simulink model "sim_tire_model"  (R2014b)
settings: Solver=ode45  StartTime=0.0  StopTime=10.0  RelTol=1e-3
settings Model: Creator=Kevin  LastModifiedBy=Kevin

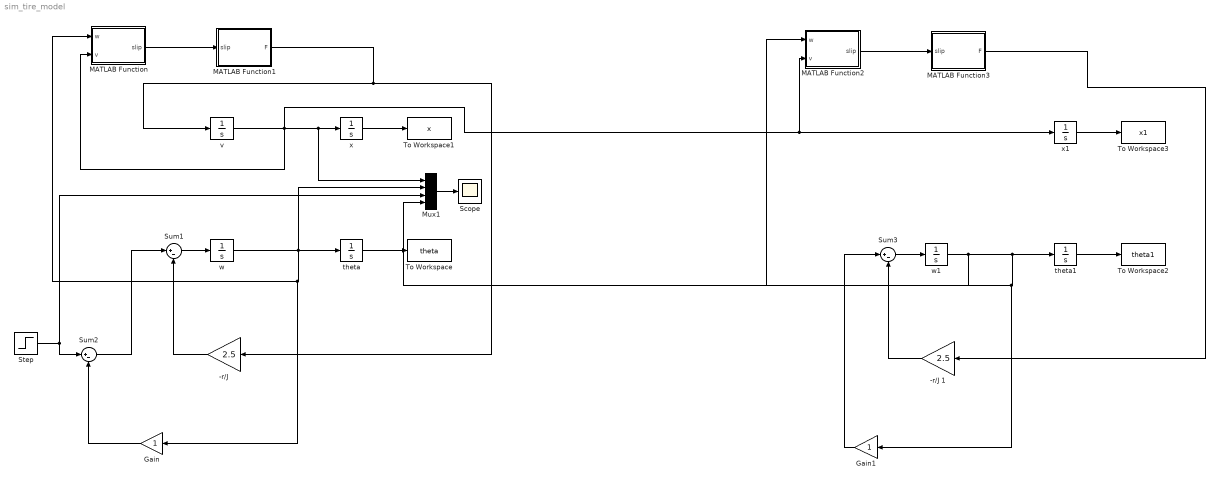
== system sim_tire_model ==
  "-r/J " : Gain  Gain=2.5
  -r/J 1 : Gain  Gain=2.5
  Gain : Gain
  Gain1 : Gain
  MATLAB Function : MATLAB Function  TreatAsAtomicUnit=on
  MATLAB Function1 : MATLAB Function  TreatAsAtomicUnit=on
  MATLAB Function2 : MATLAB Function  TreatAsAtomicUnit=on
  MATLAB Function3 : MATLAB Function  TreatAsAtomicUnit=on
  Mux1 : Mux
  Scope : Scope
      settings: ShowLegends=on
  Step : Step  Before=5  After=0  SampleTime=0
  Sum1 : Sum  Inputs=|+-
  Sum2 : Sum  Inputs=|+-
  Sum3 : Sum  Inputs=|+-
  To Workspace : ToWorkspace  VariableName=theta  SampleTime=-1
      settings: Decimation=2  Save2DSignal=2-D array (concatenate along first dimension)
  To Workspace1 : ToWorkspace  VariableName=x  SampleTime=-1
      settings: Decimation=2  Save2DSignal=2-D array (concatenate along first dimension)
  To Workspace2 : ToWorkspace  VariableName=theta1  SampleTime=-1
      settings: Decimation=2  Save2DSignal=2-D array (concatenate along first dimension)
  To Workspace3 : ToWorkspace  VariableName=x1  SampleTime=-1
      settings: Decimation=2  Save2DSignal=2-D array (concatenate along first dimension)
  theta : Integrator
  theta1 : Integrator
  "v " : Integrator
  w : Integrator
  w1 : Integrator
  x : Integrator
  x1 : Integrator
  wires:
  w/1 -> Mux1/2, Gain/1, MATLAB Function/1(w), theta/1
  "v "/1 -> MATLAB Function2/2(v), x1/1, MATLAB Function/2(v), Mux1/1, x/1
  MATLAB Function1/1(F) -> "-r/J "/1, "v "/1
  Sum1/1 -> w/1
  "-r/J "/1 -> Sum1/2
  MATLAB Function/1(slip) -> MATLAB Function1/1(slip)
  Step/1 -> Mux1/3, Sum2/1
  Sum2/1 -> Sum1/1
  Gain/1 -> Sum2/2
  theta/1 -> To Workspace/1
  x/1 -> To Workspace1/1
  MATLAB Function3/1(F) -> -r/J 1/1
  Sum3/1 -> w1/1
  -r/J 1/1 -> Sum3/2
  MATLAB Function2/1(slip) -> MATLAB Function3/1(slip)
  Gain1/1 -> Sum3/1
  theta1/1 -> To Workspace2/1
  x1/1 -> To Workspace3/1
  Mux1/1 -> Scope/1
  w1/1 -> Mux1/4, Gain1/1, MATLAB Function2/1(w), theta1/1

== matlab function sim_tire_model/MATLAB Function1 ==
  data: slip input; F output
function F = f(slip)

F = sin(2*atan((5*slip)-1*((3*slip)-atan(3*slip))));

end

== matlab function sim_tire_model/MATLAB Function ==
  data: w input; slip output; v input
function slip = f(w,v)
r = .4;

if w*r == v
    slip = 0;
else
    slip = (w*r - v) / max(w*r, v);
end

slip = floor(slip*1000)/1000;

end

== matlab function sim_tire_model/MATLAB Function2 ==
  data: w input; slip output; v input
function slip = f(w,v)
r = .4;

if w*r == v
    slip = 0;
else
    slip = (w*r - v) / max(w*r, v);
end

slip = floor(slip*1000)/1000;

end

== matlab function sim_tire_model/MATLAB Function3 ==
  data: slip input; F output
function F = f(slip)

F = sin(2*atan((5*slip)-1*((3*slip)-atan(3*slip))));

end
